simulink model "waypoint_drone_1"  (R2021a)
settings: Solver=VariableStepAuto  StartTime=0.0  StopTime=10.0  RelTol=1e-3
libraries: rllib x1
settings Model: Creator=gshetty  LastModifiedBy=gshetty

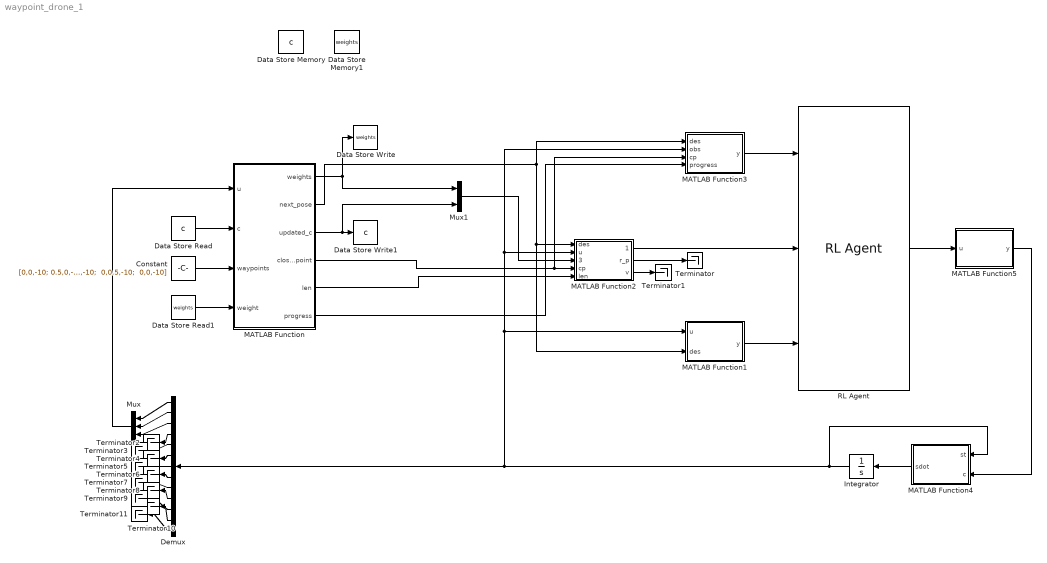
== system waypoint_drone_1 ==
  Constant : Constant  Value="[0,0,-10; 0.5,0,-10; 1,0,-10; 1.5,0,-10; 2,0,-10; 2.5,0,-10; 2.5,0.5,-10; 2.5,1,-10; 2.5,1.5,-10; 2.5,2,-10; 2.5,2.5,-10; 2,2.5,-10; 1.5,2.5,-10; 1,2.5,-10; 0.5,2.5,-10; 0,2.5,-10;  0,2,-10;  0,1.5,-10;  0,1,-10;  0,0.5,-10;  0,0,-10]"  SampleTime=-1
  Data Store Memory : DataStoreMemory  DataStoreName=c  ReadBeforeWriteMsg=warning  WriteAfterWriteMsg=warning  WriteAfterReadMsg=warning  InitialValue=1  ShowAdditionalParam=off
  Data Store Memory1 : DataStoreMemory  DataStoreName=weights  ReadBeforeWriteMsg=warning  WriteAfterWriteMsg=warning  WriteAfterReadMsg=warning  ShowAdditionalParam=off
  Data Store Read : DataStoreRead  DataStoreName=c  IndexOptions=Index vector (dialog)  Indices=1  OutputSizes=1
  Data Store Read1 : DataStoreRead  DataStoreName=weights  IndexOptions=Index vector (dialog)  Indices=1  OutputSizes=1
  Data Store Write : DataStoreWrite  DataStoreName=weights  IndexOptions=Index vector (dialog)  Indices=1  OutputSizes=1
  Data Store Write1 : DataStoreWrite  DataStoreName=c  IndexOptions=Index vector (dialog)  Indices=1  OutputSizes=1
  Demux : Demux  Outputs=13
  Integrator : Integrator
  MATLAB Function : MATLAB Function  TreatAsAtomicUnit=on
  MATLAB Function1 : MATLAB Function  TreatAsAtomicUnit=on
  MATLAB Function2 : MATLAB Function  TreatAsAtomicUnit=on
  MATLAB Function3 : MATLAB Function  TreatAsAtomicUnit=on
  MATLAB Function4 : MATLAB Function  TreatAsAtomicUnit=on
  MATLAB Function5 : MATLAB Function  TreatAsAtomicUnit=on
  Mux : Mux  Inputs=3
  Mux1 : Mux  Inputs=2
  RL Agent : rllib/RL Agent  Agent=agent  ExternalActionAsInput=off  ProvideCumRwd=off  TreatAsDirectFeedthrough=on
  Terminator{,1..11} (12 alike) : Terminator
  wires:
  RL Agent/1 -> MATLAB Function5/1(u)
  MATLAB Function3/1(y) -> RL Agent/1
  MATLAB Function2/1(reward) -> RL Agent/2
  MATLAB Function1/1(y) -> RL Agent/3
  MATLAB Function5/1(y) -> MATLAB Function4/2(c)
  MATLAB Function4/1(sdot) -> Integrator/1
  Data Store Read1/1 -> MATLAB Function/4(weight)
  Constant/1 -> MATLAB Function/3(waypoints)
  Data Store Read/1 -> MATLAB Function/2(c)
  MATLAB Function/1(weights) -> Data Store Write/1, Mux1/1
  MATLAB Function/3(updated_c) -> Mux1/2, Data Store Write1/1
  Demux/1 -> Mux/1
  Demux/2 -> Mux/2
  Demux/3 -> Mux/3
  Mux/1 -> MATLAB Function/1(u)
  Integrator/1 -> MATLAB Function3/2(obs), MATLAB Function2/2(u), MATLAB Function1/1(u), Demux/1, MATLAB Function4/1(st)
  Mux1/1 -> MATLAB Function2/3(weights)
  MATLAB Function/2(next_pose) -> MATLAB Function3/1(des), MATLAB Function1/2(des), MATLAB Function2/1(des)
  MATLAB Function/4(closest_point) -> MATLAB Function3/3(cp), MATLAB Function2/4(cp)
  MATLAB Function/5(len) -> MATLAB Function2/5(len)
  MATLAB Function/6(progress) -> MATLAB Function3/4(progress)
  MATLAB Function2/2(r_p) -> Terminator/1
  MATLAB Function2/3(v) -> Terminator1/1
  Demux/4 -> Terminator2/1
  Demux/5 -> Terminator3/1
  Demux/6 -> Terminator4/1
  Demux/7 -> Terminator5/1
  Demux/8 -> Terminator6/1
  Demux/9 -> Terminator7/1
  Demux/10 -> Terminator8/1
  Demux/11 -> Terminator9/1
  Demux/12 -> Terminator10/1
  Demux/13 -> Terminator11/1

== matlab function waypoint_drone_1/MATLAB Function1 ==
  data: u input; y output; des input
function y = fcn(u,des)
if u(3) < 0 && norm(u(1:3) - des(1:3)) < 10 && norm(u(4:6)) < 1
    y = 0;
else
    y = 1;
end

== matlab function waypoint_drone_1/MATLAB Function ==
  data: u input; weights output; c input; waypoints input; weight input; next_pose output; updated_c output; closest_point output; len output; progress output
function [weights, next_pose,updated_c,closest_point,len,progress] = fcn(u,c,waypoints,weight)
len = size(waypoints,1);
if c<len+1
    np = waypoints(c,:).';
else
    np = waypoints(len,:).';
end
if norm(u-np) < 0.03 && c<len+1
    updated_c = c + 1;
    w_v = weight + 1.0;
else
    updated_c = c;
    w_v = weight;
end
if c<=len
    np = waypoints(updated_c,:).';
else
    % w_v = 0.25*len-1;
    np = waypoints(len,:).';
end
if updated_c == 1 || updated_c == len+1
    closest_point = np;
else
    start_point = waypoints(updated_c-1,:).';
    end_point = np;
    drone_position = u;
    
    direction_vector = end_point - start_point;
    p0 = drone_position - start_point;
    t = dot(p0, direction_vector) / dot(direction_vector, direction_vector);
    t = max(0, min(1, t));
    closest_point = start_point + t * direction_vector;  
end
weights = w_v;
next_pose = [np;0.5];
progress = updated_c/len;

== matlab function waypoint_drone_1/MATLAB Function2 ==
  data: des input; u input; reward output; weights input; cp input; len input; r_p output; v output
function [reward,r_p,v] = fcn(des, u, weights,cp,len)
desired_pos = [des(1); des(2); des(3)];
% desired_v = [des(4); des(5); des(6)];
desired_vel = des(4);
% desired_o = [des(7), des(8), des(9)];
% desired_av = [des(10); des(11); des(12)];
% weights for different component of reward
w_p = weights(1);
% w_v = weights(1);
% w_o = 1.0;
% w_av = 0;
% w_collision = 10^5;
% Extract values from observation
p = [u(1); u(2); u(3)];
v = norm(u(4:6));
% o = [u(7), u(8), u(9)];
% av = [u(10); u(11); u(12)];
% calculate indivisual component of reward
% r_p =exp(-1 * abs(u(1) - desired_pos(1))) + exp(-1 * abs(u(2) - desired_pos(2))) + exp(-1 * abs(u(3) - desired_pos(3)));
r_p = w_p + (1 * exp(-1* norm(p-desired_pos)));
% r_v = w_v * exp(-1 * abs(v - desired_vel));
if weights(2) == len+1
    reward = (1 * exp(-1* norm(p-cp))) * (r_p);
else
    reward = (1 * exp(-1* norm(p-cp))) * (1 * exp(-1 * abs(v - desired_vel))) * (r_p);
    % r_v = w_v + (1 * exp(-1 * abs(v - desired_vel)));
end
% r_o = r_v;
% reward = (1 * exp(-1* norm(p-cp))) * (r_p + r_v);

== matlab function waypoint_drone_1/MATLAB Function3 ==
  data: des input; y output; obs input; cp input; progress input
function y = fcn(des, obs, cp, progress)
% Normalizing
std_pos = 10;
std_vel = 2;
std_o = pi;
std_av = 25;
norm_pos = (des(1:3)-obs(1:3))/std_pos;
norm_vel = obs(4:6)/std_vel;
norm_cp = (obs(1:3) - cp)/std_pos;
y = [norm_pos; norm_cp; des(4)-norm(obs(4:6)); norm_vel; obs(7:9)/std_o; obs(10:12)/std_av;progress];

== matlab function waypoint_drone_1/MATLAB Function4 ==
  data: st input; sdot output; c input
function sdot = fcn(st, c)
model = multirotor;
s = state(model);
s(1:13) = st;
u = control(model);
u.Roll = c(1);
u.Pitch = c(2);
u.YawRate = c(3);
u.Thrust = c(4);
e = environment(model);
sdot = derivative(model,s,u,e);

== matlab function waypoint_drone_1/MATLAB Function5 ==
  data: u input; y output
function y = fcn(u)
c1 = ((u(1) + 1) * (pi/2) / 2) - pi/4;
c2 = ((u(2) + 1) * (pi/2) / 2) - pi/4;
c3 = ((u(3) + 1) * (pi/2) / 2) - pi/4;
c4 = ((u(4) + 1) * (10) / 2) - 5;
y = [c1;c2;c3;c4];
